simulink library "LFRLIB"  (R2012b)
settings: Solver=ode45  StartTime=0.0  StopTime=10.0  RelTol=1e-3
undefined symbols (not defined in the file or in its folder): L, sysM
undefined symbols (not defined in the file): sys
libraries: simulink x1
settings Model: Creator=jmbianni  LastModifiedBy=croos

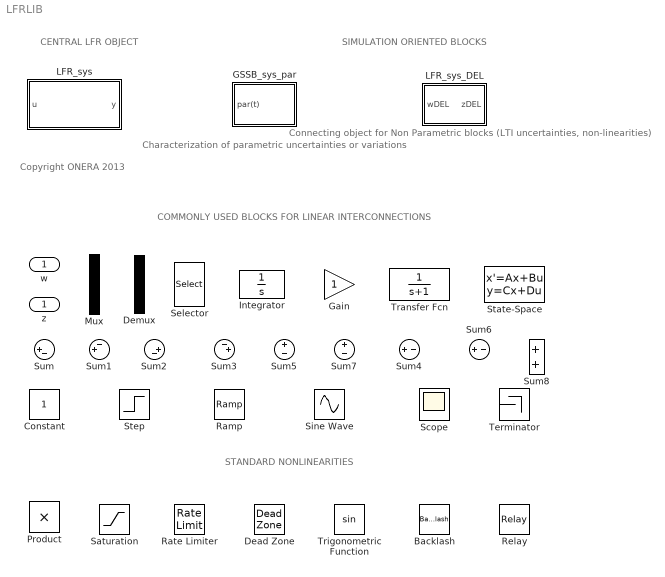
== system LFRLIB ==
  note: Copyright ONERA
      | 2013
  note: CENTRAL LFR OBJECT
  note: Characterization of parametric
      | uncertainties or variations
  note: Connecting object for Non Parametric blocks
      | (LTI uncertainties, non-linearities)
  note: SIMULATION ORIENTED BLOCKS
  note: COMMONLY USED BLOCKS FOR LINEAR INTERCONNECTIONS
  note: STANDARD NONLINEARITIES
  w : Inport
  Backlash : Backlash
  Constant : Constant
  Dead Zone : DeadZone  SaturateOnIntegerOverflow=on
  Demux : Demux  Outputs=2
  GSSB_sys_par : Subsystem  mask{sys=sys, par=par}
      mask prompts: sys "LFR-object"; par "Parameter name"
      mask init:
      | initMASKGSSP
  Gain : Gain
  Integrator : Integrator
  LFR_sys : Subsystem  mask{sys=sys}
      mask prompts: sys "LFR-object"
      mask init:
      | initMASKGSSO
  LFR_sys_DEL : Subsystem  mask{sys=sys, blkname=DEL}
      mask prompts: sys "LFR-object"; blkname "Non-Parametric block name"
      mask init:
      | initMASKGSSD
  Mux : Mux  Inputs=2
  Product : Product  RndMeth=Zero
  Ramp : simulink/Sources/Ramp  slope=1  start=0  X0=0
  Rate Limiter : RateLimiter  SampleTimeMode=inherited
  Relay : Relay
  Saturation : Saturate
  Scope : Scope
  Selector : Selector  InputPortWidth=3  IndexOptions=Index vector (dialog)  Indices=[1 3]  OutputSizes=1
  Sine Wave : Sin  SampleTime=0
  State-Space : StateSpace
  Step : Step  SampleTime=0
  Sum : Sum  Inputs=|+-
  Sum1 : Sum  Inputs=-+|
  Sum2 : Sum  Inputs=|+-
  Sum3 : Sum  Inputs=-+|
  Sum{4..7} (4 alike) : Sum  Inputs=+|-
  Sum8 : Sum
  Terminator : Terminator
  Transfer Fcn : TransferFcn  Denominator=[1 1]
  Trigonometric Function : Trigonometry
  z : Outport

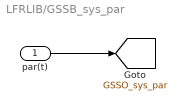
== system LFRLIB/GSSB_sys_par ==
  par(t) : Inport
  tag scope: GSSO_sys_par=global
  wires:
  par(t)/1 -> [GSSO_sys_par]

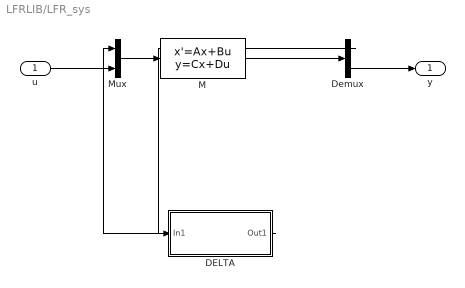
== system LFRLIB/LFR_sys ==
  u : Inport
  DELTA : Subsystem
  Demux : Demux  Outputs=dimDemux
  M : StateSpace  A=sysM.a  B=sysM.b  C=sysM.c  D=sysM.d
  Mux : Mux  Inputs=dimMux
  y : Outport
  wires:
  M/1 -> Demux/1
  Demux/2 -> y/1
  u/1 -> Mux/2
  Mux/1 -> M/1
  Demux/1 -> DELTA/1(In1)
  DELTA/1(Out1) -> Mux/1

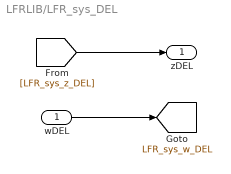
== system LFRLIB/LFR_sys_DEL ==
  wDEL : Inport
  zDEL : Outport
  tag scope: LFR_sys_w_DEL=global
  wires:
  wDEL/1 -> [LFR_sys_w_DEL]
  [LFR_sys_z_DEL] -> zDEL/1

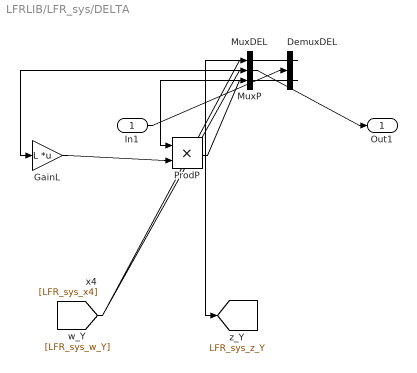
== system LFRLIB/LFR_sys/DELTA ==
  In1 : Inport
  DemuxDEL : Demux  Outputs=[ 5 3]
  GainL : Gain  Gain=L  Multiplication=Matrix(K*u)
  MuxDEL : Mux  Inputs=[ 3 3]
  MuxP : Mux  Inputs=1
  ProdP : Product  RndMeth=Zero
  Out1 : Outport
  tag scope: LFR_sys_z_Y=global
  wires:
  In1/1 -> DemuxDEL/1
  MuxDEL/1 -> Out1/1
  DemuxDEL/1 -> [LFR_sys_z_Y]
  [LFR_sys_w_Y] -> MuxDEL/1
  [LFR_sys_x4] -> MuxP/1
  MuxP/1 -> GainL/1
  DemuxDEL/2 -> ProdP/1
  GainL/1 -> ProdP/2
  ProdP/1 -> MuxDEL/2
